simulink model "assignment1_voo"  (R2022b)
settings: Solver=FixedStepAuto  StartTime=0.0  StopTime=1  FixedStep=1e-3  RelTol=1e-3  EnableMultiTasking=on
undefined symbols (not defined in the file): D10, D11, D12, D2, D4, D5, D7, D8, D9, PTA0, PTA2, PTB23, PTB9, PTC3, PTC4, PTD0, PTD2, PTD3
libraries: frdmk64flib x9
settings Model: ExtModeTrigDuration=5  Creator=tammyz  LastModifiedBy=tammyz
settings SolverCC: AlgebraicLoopSolver=TrustRegion
settings OptimizationCC: EnhancedBackFolding=on  PassReuseOutputArgsAs=Individual arguments  ZeroExternalMemoryAtStartup=off  ZeroInternalMemoryAtStartup=off  MaxStackSize=64  OptimizeBlockOrder=speed  DifferentSizesBufferReuse=on  OptimizationCustomize=off  EfficientTunableParamExpr=on
settings DebuggingCC: ParameterTunabilityLossMsg=error  UnconnectedInputMsg=warning  UnconnectedOutputMsg=warning  UnconnectedLineMsg=warning  SFMachineParentedDataDiag=warning
settings HardwareCC: ProdBitPerPointer=32  ProdBitPerSizeT=32  ProdBitPerPtrDiffT=32  ProdLargestAtomicInteger=Long  ProdLargestAtomicFloat=Double  ProdWordSize=32  ProdHWDeviceType=ARM Compatible->ARM Cortex
settings ModelReferenceCC: EnableRefExpFcnMdlSchedulingChecks=on
settings SFSimCC: MATLABDynamicMemAlloc=off
settings RTWCC: Description=Embedded Coder  SystemTargetFile=ert.tlc  HardwareBoard=NXP FRDM-K64F  TLCOptions="-aInlineSetEventsForThisBaseRateFcn=TLC_FALSE -aSuppressMultiTaskScheduler=TLC_FALSE  -aRateBasedStepFcn=0"  TemplateMakefile=ert_default_tmf  Toolchain=GNU Tools for ARM Embedded Processors
settings CodeAppCC: ForceParamTrailComments=on  IgnoreCustomStorageClasses=off  OperatorAnnotations=on  SimulinkDataObjDesc=on  SFDataObjDesc=on  InsertBlockDesc=on

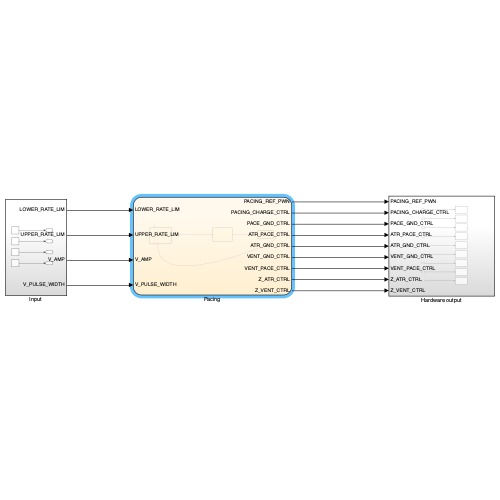
[thumbnail: Simulink's stored preview of the top-level diagram]
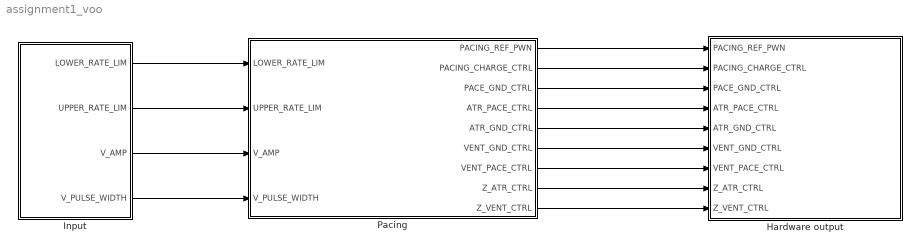
== system assignment1_voo ==
  Hardware output : Subsystem
  Input : Subsystem
  Pacing : Stateflow chart  TreatAsAtomicUnit=on
  wires:
  Pacing/1(PACING_REF_PWN) -> Hardware output/1(PACING_REF_PWN)
  Pacing/2(PACING_CHARGE_CTRL) -> Hardware output/2(PACING_CHARGE_CTRL)
  Pacing/3(PACE_GND_CTRL) -> Hardware output/3(PACE_GND_CTRL)
  Pacing/4(ATR_PACE_CTRL) -> Hardware output/4(ATR_PACE_CTRL)
  Pacing/5(ATR_GND_CTRL) -> Hardware output/5(ATR_GND_CTRL)
  Pacing/6(VENT_GND_CTRL) -> Hardware output/6(VENT_GND_CTRL)
  Pacing/7(VENT_PACE_CTRL) -> Hardware output/7(VENT_PACE_CTRL)
  Pacing/8(Z_ATR_CTRL) -> Hardware output/8(Z_ATR_CTRL)
  Pacing/9(Z_VENT_CTRL) -> Hardware output/9(Z_VENT_CTRL)
  Input/4(V_PULSE_WIDTH) -> Pacing/4(V_PULSE_WIDTH)
  Input/3(V_AMP) -> Pacing/3(V_AMP)
  Input/1(LOWER_RATE_LIM) -> Pacing/1(LOWER_RATE_LIM)
  Input/2(UPPER_RATE_LIM) -> Pacing/2(UPPER_RATE_LIM)

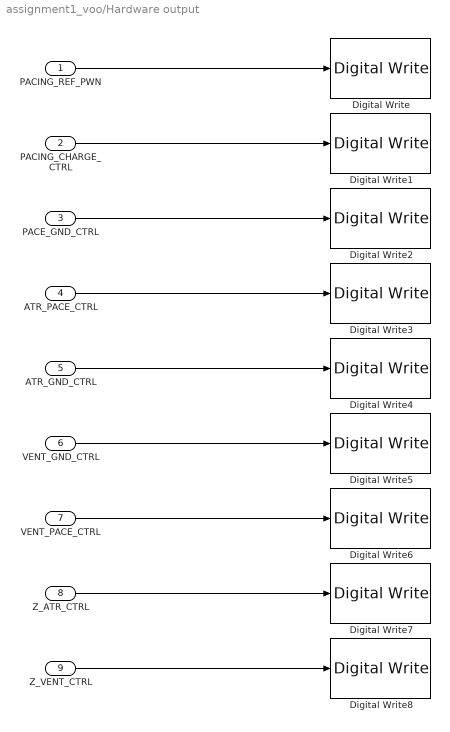
== system assignment1_voo/Hardware output ==
  PACING_REF_PWN : Inport
  PACING_CHARGE_CTRL : Inport  Port=2
  PACE_GND_CTRL : Inport  Port=3
  ATR_PACE_CTRL : Inport  Port=4
  ATR_GND_CTRL : Inport  Port=5
  VENT_GND_CTRL : Inport  Port=6
  VENT_PACE_CTRL : Inport  Port=7
  Z_ATR_CTRL : Inport  Port=8
  Z_VENT_CTRL : Inport  Port=9
  Digital Write : frdmk64flib/Digital Write  Whichpin=PTA2 (D5)
  Digital Write1 : frdmk64flib/Digital Write  Whichpin=PTB9 (D2)
  Digital Write2 : frdmk64flib/Digital Write  Whichpin=PTD0 (D10)
  Digital Write3 : frdmk64flib/Digital Write  Whichpin=PTA0 (D8)
  Digital Write4 : frdmk64flib/Digital Write  Whichpin=PTD2 (D11)
  Digital Write5 : frdmk64flib/Digital Write  Whichpin=PTD3 (D12)
  Digital Write6 : frdmk64flib/Digital Write  Whichpin=PTC4 (D9)
  Digital Write7 : frdmk64flib/Digital Write  Whichpin=PTB23 (D4)
  Digital Write8 : frdmk64flib/Digital Write  Whichpin=PTC3 (D7)
  wires:
  PACING_REF_PWN/1 -> Digital Write/1
  PACING_CHARGE_CTRL/1 -> Digital Write1/1
  PACE_GND_CTRL/1 -> Digital Write2/1
  ATR_PACE_CTRL/1 -> Digital Write3/1
  ATR_GND_CTRL/1 -> Digital Write4/1
  VENT_GND_CTRL/1 -> Digital Write5/1
  VENT_PACE_CTRL/1 -> Digital Write6/1
  Z_ATR_CTRL/1 -> Digital Write7/1
  Z_VENT_CTRL/1 -> Digital Write8/1

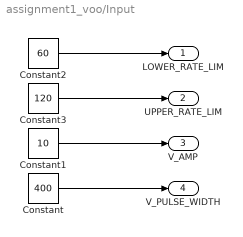
== system assignment1_voo/Input ==
  Constant : Constant  Value=400
  Constant1 : Constant  Value=10
  Constant2 : Constant  Value=60
  Constant3 : Constant  Value=120
  LOWER_RATE_LIM : Outport
  UPPER_RATE_LIM : Outport  Port=2
  V_AMP : Outport  Port=3
  V_PULSE_WIDTH : Outport  Port=4
  wires:
  Constant/1 -> V_PULSE_WIDTH/1
  Constant1/1 -> V_AMP/1
  Constant3/1 -> UPPER_RATE_LIM/1
  Constant2/1 -> LOWER_RATE_LIM/1

== stateflow chart assignment1_voo/Pacing ==
  state CHARGING_C22
    PACING_CHARGE_CTRL = true
    PACE_GND_CTRL = true
    ATR_PACE_CTRL = false
    ATR_GND_CTRL = false
    VENT_PACE_CTRL = false
    VENT_GND_CTRL = true
    PACING_REF_PWN = V_AMP/5
    Z_ATR_CTRL = false
    Z_VENT_CTRL = false
  state DISCHARGING
    PACING_CHARGE_CTRL = false
    PACE_GND_CTRL = true
    ATR_GND_CTRL = false
    VENT_GND_CTRL = false
  state INTERMEDIATE
    VENT_PACE_CTRL = true
  (default) -> CHARGING_C22
  CHARGING_C22 -> DISCHARGING : after(V_PULSE_WIDTH, msec){PACING_CHARGE_CTRL = false}
  DISCHARGING -> INTERMEDIATE
  INTERMEDIATE -> CHARGING_C22 : after(LOWER_RATE_LIM, msec)
  data: PACING_REF_PWN output double; PACING_CHARGE_CTRL output boolean; PACE_GND_CTRL output boolean; LOWER_RATE_LIM input double; UPPER_RATE_LIM input double; V_AMP input double; V_PULSE_WIDTH input double; ATR_PACE_CTRL output boolean; ATR_GND_CTRL output boolean; VENT_GND_CTRL output boolean; VENT_PACE_CTRL output boolean; Z_ATR_CTRL output boolean; Z_VENT_CTRL output boolean
